simulink model "symulacja_old"  (R2021b)
settings: Solver=VariableStepAuto  StartTime=0.0  StopTime=10.0  MaxStep=0.01  RelTol=1e-3
values from neighbouring files (symbols this model uses):
  A = [ 0     1         0         0 ... (first row only)    [lab3.m]
  B = [0; 1/M; 0; 1/(M*L)]    [lab3.m]
  C = diag([1 1 1 1])    [lab3.m]
  D = zeros(4, 1)    [lab3.m]
  K = lqr(A, B, Q, R)    [lab3.m]
  x0 = [0; 0; 0; 0]    [lab3.m]
  y0 = [2; 0; 0; 0]    [lab3.m]
settings Model: Creator=maciejholodniuk  LastModifiedBy=maciejholodniuk
settings DebuggingCC: UnconnectedInputMsg=none  UnconnectedOutputMsg=none  UnconnectedLineMsg=none
settings ModelReferenceCC: EnableRefExpFcnMdlSchedulingChecks=off
settings RTWCC: DLArmComputeVersion=20.02.1

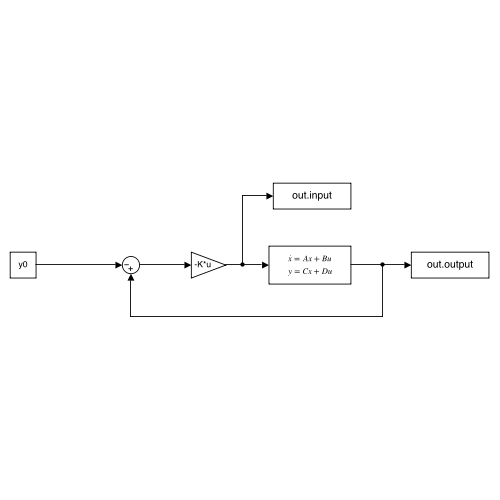
[thumbnail: Simulink's stored preview of the top-level diagram]
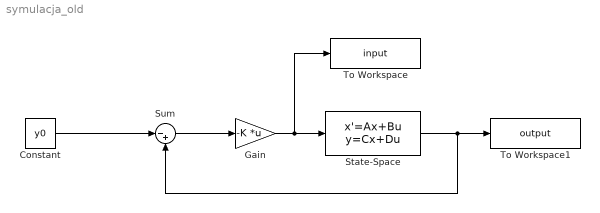
== system symulacja_old ==
  Constant : Constant  Value=y0
  Gain : Gain  Gain=-K  Multiplication=Matrix(K*u)
  State-Space : StateSpace  A=A  B=B  C=C  D=D  InitialCondition=x0
  Sum : Sum  Inputs=|-+
  To Workspace : ToWorkspace  VariableName=input  SaveFormat=Timeseries  SampleTime=-1
  To Workspace1 : ToWorkspace  VariableName=output  SaveFormat=Timeseries  SampleTime=-1
  wires:
  Sum/1 -> Gain/1
  Gain/1 -> To Workspace/1, State-Space/1
  State-Space/1 -> Sum/2, To Workspace1/1
  Constant/1 -> Sum/1
